simulink model "reg_dsf"  (R2017a)
settings: Solver=ode45  StartTime=0.0  StopTime=5.625  RelTol=1e-3  EnableMultiTasking=on
values from neighbouring files (symbols this model uses):
  A = [0 1 0; -4 -.4 40; 0 0 -4]    [hw8.m]
  B = [0;0;2]    [hw8.m]
  K = place(phi, gamma, zPoles)    [hw8.m]
  T = min(pi/beta_max,Ts/(20*n))    [hw8.m]
  x0 = [0.34;0;0]    [hw8.m]
settings Model: Creator=rjv  LastModifiedBy=noah
settings DataIOCC: LimitDataPoints=on  SaveFormat=Array
settings OptimizationCC: LifeSpan=inf
settings DebuggingCC: SFUnexpectedBacktrackingDiag=warning  SFNoUnconditionalDefaultTransitionDiag=warning  SFExecutionAtInitializationDiag=none
settings HardwareCC: ProdBitPerPointer=32  ProdBitPerSizeT=32  ProdBitPerPtrDiffT=32  ProdLargestAtomicFloat=None  ProdIntDivRoundTo=Undefined  ProdEndianess=Unspecified  ProdWordSize=32  ProdHWDeviceType=32-bit Generic
settings ModelReferenceCC: PropagateSignalLabelsOutOfModel=off
settings GRTTargetCC: TargetLangStandard=C89/C90 (ANSI)  GeneratePreprocessorConditionals=Disable all
settings ConfigComp: CovMetricSettings=dw  CovHtmlReporting=on  CovSaveCumulativeToWorkspaceVar=on  CovSaveSingleToWorkspaceVar=on  CovExternalEMLEnable=off

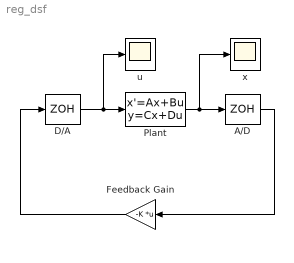
== system reg_dsf ==
  A/D : ZeroOrderHold  SampleTime=T
  D/A : ZeroOrderHold  SampleTime=T
  Feedback Gain : Gain  Gain=-K  Multiplication=Matrix(K*u)
  Plant : StateSpace  A=A  B=B  C=eye(length(A))  D=zeros(length(A),min(size((B))))  X0=x0
  u : Scope
  x : Scope
  wires:
  Plant/1 -> A/D/1, x/1
  D/A/1 -> u/1, Plant/1
  A/D/1 -> Feedback Gain/1
  Feedback Gain/1 -> D/A/1
